simulink model "digi_modu"  (R2019b)
settings: Solver=VariableStepAuto  StartTime=0.0  StopTime=1  RelTol=1e-3
settings Model: Creator=yango  LastModifiedBy=yango

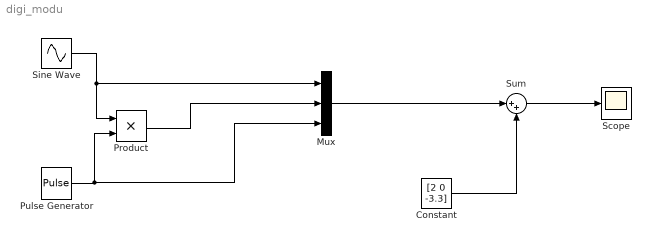
== system digi_modu ==
  Constant : Constant  Value=[2 0 -3.3]
  Mux : Mux  Inputs=3
  Product : Product
  Pulse Generator : DiscretePulseGenerator  PulseType=Time based  Period=0.02  PulseWidth=50
  Scope : Scope
  Sine Wave : Sin  Frequency=2*pi  SampleTime=0
  Sum : Sum  Inputs=|++  SaturateOnIntegerOverflow=on
  wires:
  Sine Wave/1 -> Mux/1, Product/1
  Pulse Generator/1 -> Mux/3, Product/2
  Constant/1 -> Sum/2
  Mux/1 -> Sum/1
  Sum/1 -> Scope/1
  Product/1 -> Mux/2
